simulink model "jacobian_pseudo_inverse_2018b"  (R2019b)
settings: Solver=VariableStepAuto  StartTime=0.0  StopTime=4  RelTol=1e-3
undefined symbols (not defined in the file or in its folder): DiscIntNeverNeededParam, q0, Tc
settings Model: Creator=GA  LastModifiedBy=GA
settings SFSimCC: CustomCodeUndefinedFunction=UseInterfaceOnly

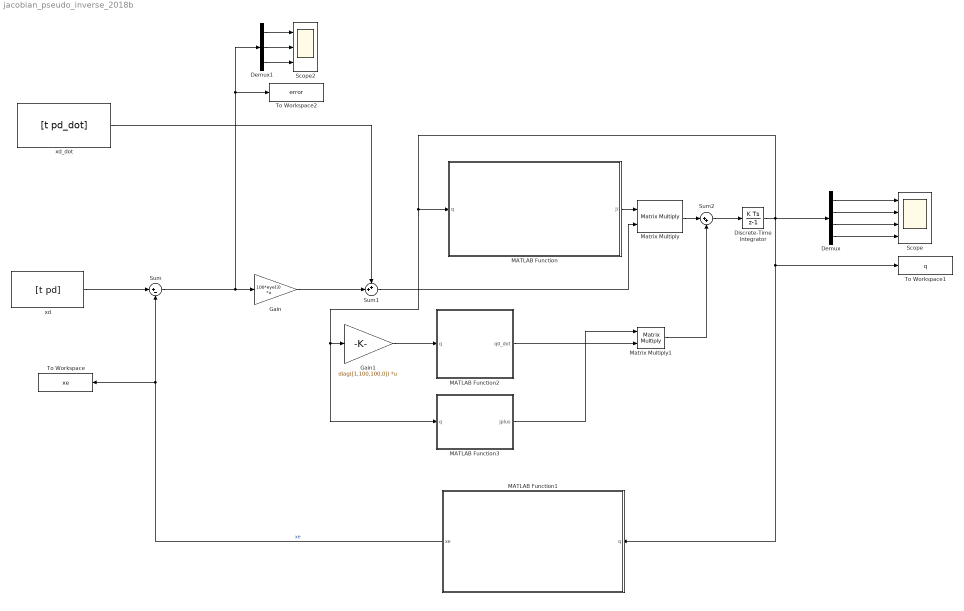
== system jacobian_pseudo_inverse_2018b ==
  Demux : Demux
  Demux1 : Demux  Outputs=3
  Discrete-Time Integrator : DiscreteIntegrator  gainval=1  InitialCondition=q0  SampleTime=Tc  ICPrevOutput=DiscIntNeverNeededParam  ICPrevScaledInput=DiscIntNeverNeededParam
  Gain : Gain  Gain=100*eye(3)  Multiplication=Matrix(K*u)
  Gain1 : Gain  Gain=diag([1,100,100,0])  Multiplication=Matrix(K*u)
  MATLAB Function : MATLAB Function  TreatAsAtomicUnit=on
  MATLAB Function1 : MATLAB Function  TreatAsAtomicUnit=on
  MATLAB Function2 : MATLAB Function  TreatAsAtomicUnit=on
  MATLAB Function3 : MATLAB Function  TreatAsAtomicUnit=on
  Matrix Multiply : Product  Multiplication=Matrix(*)
  Matrix Multiply1 : Product  Multiplication=Matrix(*)
  Scope : Scope  NumInputPorts=4
  Scope2 : Scope  NumInputPorts=3
  Sum : Sum  Inputs=|+-
  Sum1 : Sum  Inputs=++|
  Sum2 : Sum  Inputs=|++
  To Workspace : ToWorkspace  VariableName=xe  SaveFormat=Timeseries  SampleTime=-1
  To Workspace1 : ToWorkspace  VariableName=q  SaveFormat=Timeseries  SampleTime=-1
  To Workspace2 : ToWorkspace  VariableName=error  SaveFormat=Timeseries  SampleTime=Tc
  xd : FromWorkspace  VariableName=[t pd]  SampleTime=Tc
  xd_dot : FromWorkspace  VariableName=[t pd_dot]  SampleTime=Tc
  wires:
  MATLAB Function1/1(xe) -> To Workspace/1, Sum/2  "xe"
  Gain/1 -> Sum1/2
  Discrete-Time Integrator/1 -> MATLAB Function1/1(q), To Workspace1/1, MATLAB Function3/1(q), Gain1/1, MATLAB Function/1(q), Demux/1
  Sum1/1 -> Matrix Multiply/2
  Demux/3 -> Scope/3
  Demux/2 -> Scope/2
  xd_dot/1 -> Sum1/1
  Demux1/1 -> Scope2/1
  Demux/1 -> Scope/1
  MATLAB Function/1(ji) -> Matrix Multiply/1
  Demux1/3 -> Scope2/3
  xd/1 -> Sum/1
  Sum/1 -> To Workspace2/1, Demux1/1, Gain/1
  Demux1/2 -> Scope2/2
  Gain1/1 -> MATLAB Function2/1(q)
  Matrix Multiply/1 -> Sum2/1
  Matrix Multiply1/1 -> Sum2/2
  Sum2/1 -> Discrete-Time Integrator/1
  MATLAB Function3/1(jplus) -> Matrix Multiply1/1
  MATLAB Function2/1(q0_dot) -> Matrix Multiply1/2
  Demux/4 -> Scope/4

== matlab function jacobian_pseudo_inverse_2018b/MATLAB Function1 ==
  data: q input; xe output
function xe = non_linear_function(q)
a1 = 0.5;
a2 = 0.5;
d0 = 1;
xe = zeros(3,1);
xe(1,:) = a1*cos(q(1))+a2*cos(q(1)+q(2));
xe(2,:) = a1*sin(q(1))+a2*sin(q(1)+q(2));
xe(3,:) = d0 - q(3);
% xe(4,:) = q(1)+q(2);

== matlab function jacobian_pseudo_inverse_2018b/MATLAB Function ==
  data: q input; ji output
function ji = jacobian_pseudo_inverse(q)
    
a1 = 0.5;
a2 = 0.5;

j = zeros(3,4);
j(1,1) = -a1*sin(q(1))-a2*sin(q(1)+q(2));
j(1,2) = -a2*sin(q(1)+q(2));
j(2,1) = a1*cos(q(1))+a2*cos(q(1)+q(2));
j(2,2) = a2*cos(q(1)+q(2));
j(3,3) = -1;
% j(4,1) = 1;
% j(4,2) = 1;
% j(4,4) = 1;
ji = j'*inv(j*j');

== matlab function jacobian_pseudo_inverse_2018b/MATLAB Function2 ==
  data: q input; q0_dot output
function q0_dot = constraint_function(q)
q0_dot = zeros(4,1);
q0_dot(1) = -q(1)/(pi^2);
q0_dot(2) = -(q(2)+(pi/8))/((3*pi/4)^2);
q0_dot(3) = -(q(3)-0.625)/((.75)^2);

== matlab function jacobian_pseudo_inverse_2018b/MATLAB Function3 ==
  data: q input; jplus output
function jplus = constraint_jacobian(q)

a1 = 0.5;
a2 = 0.5;

j = zeros(3,4);
j(1,1) = -a1*sin(q(1))-a2*sin(q(1)+q(2));
j(1,2) = -a2*sin(q(1)+q(2));
j(2,1) = a1*cos(q(1))+a2*cos(q(1)+q(2));
j(2,2) = a2*cos(q(1)+q(2));
j(3,3) = -1;
% j(4,1) = 1;
% j(4,2) = 1;
% j(4,4) = 1;
jplus = eye(4)-j'*inv(j*j')*j;
